simulink model "Controle_UDP_0104"  (R2014a)
settings: Solver=ode45  StartTime=0.0  StopTime=inf  RelTol=1e-3
values from neighbouring files (symbols this model uses):
  in1 = [ 10 10 25 30 0 ] * pi / 180    [data_ACS_HIL.m]
  in2 = [ 0 10 10 30 0 ] * pi / 180    [data_ACS_HIL.m]
  in3 = [ 45 -30 30 30 0 ] * pi / 180    [data_ACS_HIL.m]
  Ixx = I( 1, 1 )    [data_ACS_HIL.m]
  Iyy = I( 2, 2 )    [data_ACS_HIL.m]
  Izz = I( 3, 3 )    [data_ACS_HIL.m]
  J1 = I1 + 3e-06    (= 0.000627567)    [data_ACS_HIL.m]
  J2 = I2 + 3e-06    (= 0.000627567)    [data_ACS_HIL.m]
  J3 = I3 + 3e-06    (= 0.000627567)    [data_ACS_HIL.m]
  Kpx = vp * (wn^2) * Ixx    [data_ACS_HIL.m]
  Kpy = vp * (wn^2) * Iyy    [data_ACS_HIL.m]
  Kpz = vp * (wn^2) * Izz    [data_ACS_HIL.m]
  Krx = vr * 2 * Ixx * wn * qsi    [data_ACS_HIL.m]
  Kry = vr * 2 * Iyy * wn * qsi    [data_ACS_HIL.m]
  Krz = vr * 2 * Izz * wn * qsi    [data_ACS_HIL.m]
  Wx0 = [mW0 0]    [data_ACS_HIL.m]
  Wy0 = [mW0 0]    [data_ACS_HIL.m]
  Wz0 = [mW0 0]    [data_ACS_HIL.m]
libraries: aerolibconvert2 x4, simulink x3, etargetslib x2, instrumentlib x2, xpcutilitieslib x1, slrtlib x1, rtwinlib x1
settings Model: Creator=mayar_000  LastModifiedBy=IMA4BRAZIL
settings DataIOCC: SignalLoggingSaveFormat=ModelDataLogs
settings DebuggingCC: MultiTaskDSMMsg=warning  MultiTaskCondExecSysMsg=none  IntegerOverflowMsg=none  ParameterOverflowMsg=none
settings RTWCC: IncludeERTFirstTime=on

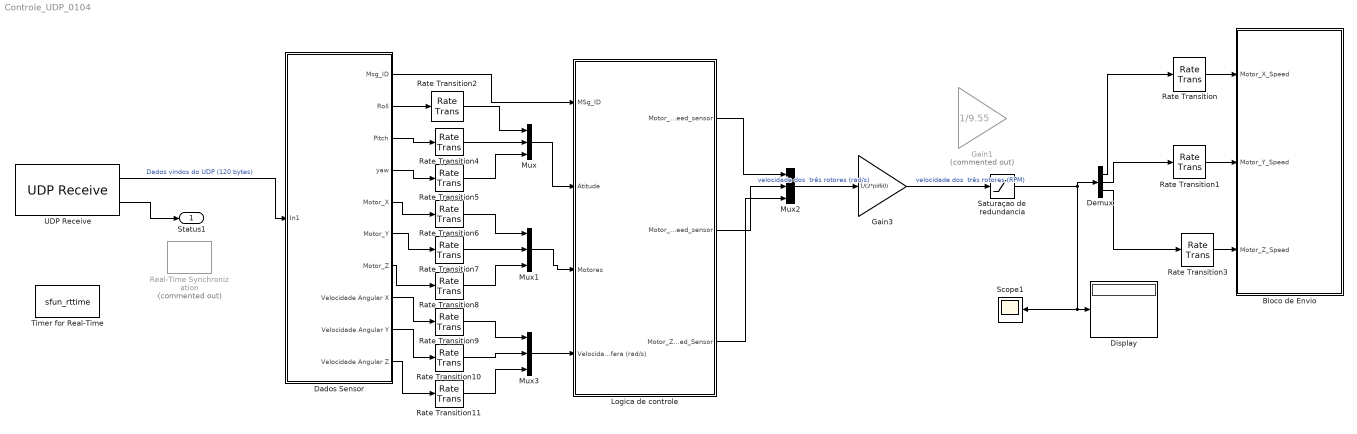
== system Controle_UDP_0104 ==
  Bloco de Envio : Subsystem
      mask Display:
      | port_label('input',1,'\Omega_x','texmode','on')
      | port_label('input',2,'\Omega_y','texmode','on')
      | port_label('input',3,'\Omega_z','texmode','on')
  Dados Sensor : Subsystem
  Demux : Demux  Outputs=3
  Display : Display
  Gain1 : Gain  Commented=on  Gain=1/9.55  SaturateOnIntegerOverflow=on
  Gain3 : Gain  Gain=1/(2*pi/60)
  Logica de controle : Subsystem
  Mux{,1..3} (4 alike) : Mux  Inputs=3
  Rate Transition{,1..11} (12 alike) : RateTransition  OutPortSampleTime=t
  Real-Time Synchronization : rtwinlib/Real-Time Synchronization  Commented=on  SampleTime=0.1  MaxMissedTicks=20  ShowMissedTicks=off  YieldWhenWaiting=off
  Saturaçao de redundancia : Saturate  UpperLimit=4000  LowerLimit=-4000
  Scope1 : Scope
      settings: YMin=-10000  YMax=10000
  Timer for Real-Time : S-Function  FunctionName=sfun_rttime  Parameters=1  EnableBusSupport=off
  UDP Receive : instrumentlib/UDP Receive  Host=172.16.0.62  Port=35204  LocalPort=35204  DataSize=120  EnableBlockingMode=off  Timeout=50  SampleTime=0.25  DataType=uint8  ByteOrder=BigEndian
  Status1 : Outport
  wires:
  UDP Receive/2 -> Status1/1
  UDP Receive/1 -> Dados Sensor/1(In1)  "Dados vindos do UDP (120 bytes)"
  Rate Transition/1 -> Bloco de Envio/1(Motor_X_Speed)
  Rate Transition1/1 -> Bloco de Envio/2(Motor_Y_Speed)
  Demux/1 -> Rate Transition/1
  Demux/2 -> Rate Transition1/1
  Demux/3 -> Rate Transition3/1
  Rate Transition3/1 -> Bloco de Envio/3(Motor_Z_Speed)
  Dados Sensor/1(Msg_ID) -> Logica de controle/1(MSg_ID)
  Mux/1 -> Logica de controle/2(Atitude)
  Mux1/1 -> Logica de controle/3(Motores)
  Logica de controle/1(Motor_X_Speed_sensor) -> Mux2/1
  Logica de controle/2(Motor_Y_Speed_sensor) -> Mux2/2
  Logica de controle/3(Motor_Z_Speed_Sensor) -> Mux2/3
  Dados Sensor/2(Roll) -> Rate Transition2/1
  Dados Sensor/3(Pitch) -> Rate Transition4/1
  Dados Sensor/4(yaw) -> Rate Transition5/1
  Dados Sensor/7(Motor_Z) -> Rate Transition8/1
  Dados Sensor/6(Motor_Y) -> Rate Transition7/1
  Dados Sensor/5(Motor_X) -> Rate Transition6/1
  Rate Transition2/1 -> Mux/1
  Rate Transition4/1 -> Mux/2
  Rate Transition5/1 -> Mux/3
  Rate Transition6/1 -> Mux1/1
  Rate Transition7/1 -> Mux1/2
  Rate Transition8/1 -> Mux1/3
  Saturaçao de redundancia/1 -> Demux/1, Scope1/1, Display/1
  Mux2/1 -> Gain3/1  "velocidade dos  três rotores (rad/s)"
  Gain3/1 -> Saturaçao de redundancia/1  "velocidade dos  três rotores (RPM)"
  Dados Sensor/8(Velocidade Angular X) -> Rate Transition9/1
  Dados Sensor/9(Velocidade Angular Y) -> Rate Transition10/1
  Dados Sensor/10(Velocidade Angular Z) -> Rate Transition11/1
  Mux3/1 -> Logica de controle/4(Velocidade Angular da Esfera (rad/s))
  Rate Transition9/1 -> Mux3/1
  Rate Transition10/1 -> Mux3/2
  Rate Transition11/1 -> Mux3/3

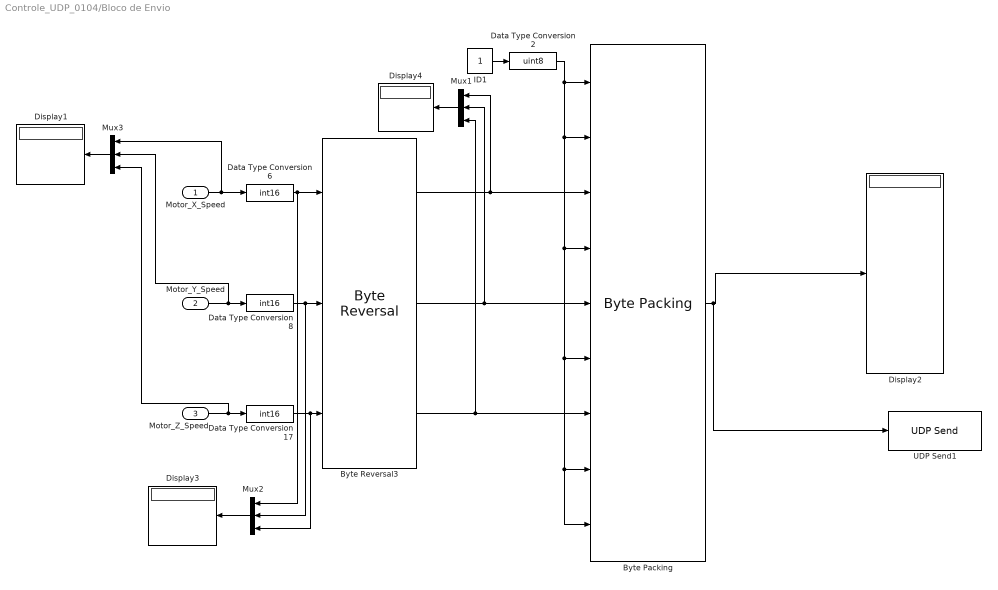
== system Controle_UDP_0104/Bloco de Envio ==
  Motor_X_Speed : Inport
  Motor_Y_Speed : Inport  Port=2
  Motor_Z_Speed : Inport  Port=3
  "Byte Packing " : xpcutilitieslib/Byte Packing   MaskPackedDataType=uint8  MaskUnpackedDataTypes={'uint8','uint8','int16','uint8','int16','uint8','int16','uint8', 'uint8'}  MaskAlignment=1
  Byte Reversal3 : etargetslib/Byte Reversal  numInp=3
  Data Type Conversion17 : DataTypeConversion  OutDataTypeStr=int16  SaturateOnIntegerOverflow=on
  Data Type Conversion2 : DataTypeConversion  OutDataTypeStr=uint8  SaturateOnIntegerOverflow=on
  Data Type Conversion6 : DataTypeConversion  OutDataTypeStr=int16  SaturateOnIntegerOverflow=on
  Data Type Conversion8 : DataTypeConversion  OutDataTypeStr=int16  SaturateOnIntegerOverflow=on
  Display{1..4} (4 alike) : Display
      Display3 settings: Format=hex (Stored Integer)
      Display4 settings: Format=hex (Stored Integer)
  ID1 : Constant  OutDataTypeStr=uint8
  Mux1 : Mux  Inputs=3
  Mux2 : Mux  Inputs=3
  Mux3 : Mux  Inputs=3
  UDP Send1 : instrumentlib/UDP Send  Host=172.16.0.62  Port=35308  LocalPort=-1  EnableBlockingMode=off  ByteOrder=LittleEndian
  wires:
  Motor_Y_Speed/1 -> Mux3/2, Data Type Conversion8/1
  Data Type Conversion6/1 -> Mux2/1, Byte Reversal3/1
  Motor_X_Speed/1 -> Mux3/1, Data Type Conversion6/1
  "Byte Packing "/1 -> Display2/1, UDP Send1/1
  Data Type Conversion8/1 -> Mux2/2, Byte Reversal3/2
  Data Type Conversion17/1 -> Mux2/3, Byte Reversal3/3
  Byte Reversal3/2 -> Mux1/2, "Byte Packing "/5
  Data Type Conversion2/1 -> "Byte Packing "/9, "Byte Packing "/8, "Byte Packing "/6, "Byte Packing "/4, "Byte Packing "/2, "Byte Packing "/1
  ID1/1 -> Data Type Conversion2/1
  Byte Reversal3/1 -> Mux1/1, "Byte Packing "/3
  Mux3/1 -> Display1/1
  Mux1/1 -> Display4/1
  Byte Reversal3/3 -> Mux1/3, "Byte Packing "/7
  Motor_Z_Speed/1 -> Mux3/3, Data Type Conversion17/1
  Mux2/1 -> Display3/1

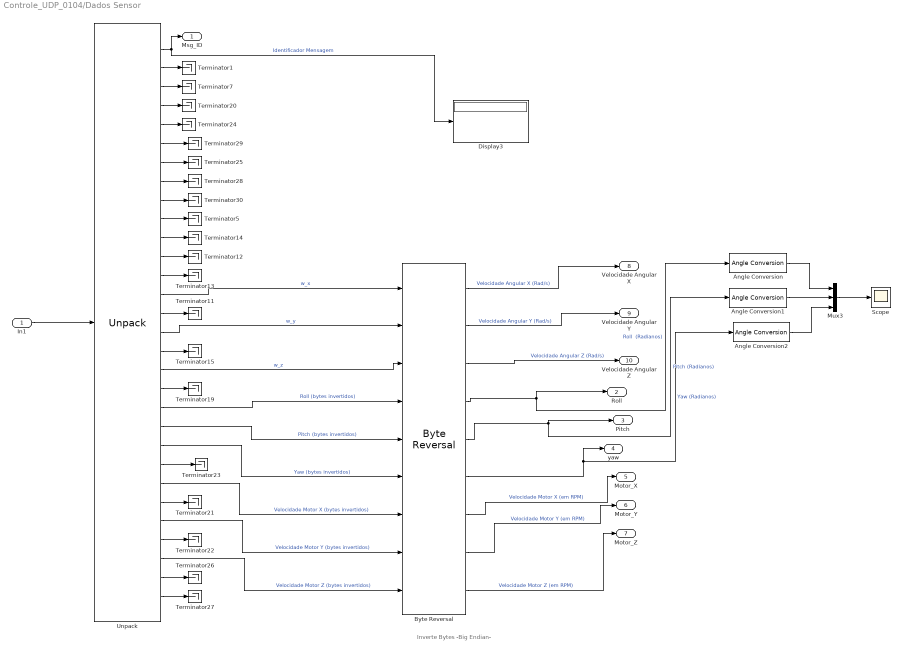
== system Controle_UDP_0104/Dados Sensor ==
  note: Inverte Bytes
      | -Big Endian-
  In1 : Inport
  Angle Conversion : aerolibconvert2/Angle Conversion  IU=rad  OU=deg
  Angle Conversion1 : aerolibconvert2/Angle Conversion  IU=rad  OU=deg
  Angle Conversion2 : aerolibconvert2/Angle Conversion  IU=rad  OU=deg
  Byte Reversal : etargetslib/Byte Reversal  numInp=9
  Display3 : Display
  Mux3 : Mux  Inputs=3
  Scope : Scope
      settings: YMin=-10  YMax=100  SaveName=ScopeData2
  Terminator{1,5,7,11..15,19..30} (20 alike) : Terminator
  Unpack : slrtlib/UDP/Unpack   dimensions={[1,1],[1,1],[1,1],[1,1],[1,1],[1,1],[1,1],[1,1],[1,1],[1,1],[1,1],[1,1],[1,1],[1,1],[1,1],[1,1],[1,1],[1,1],[1,1],[1,1],[1,1],[1,1],[1,4],[1,1],[1,1],[1,1],[1,1],[1,1],[1,1],[1,1]}  datatypes={'uint8','single','uint32','single','uint32','single','uint32','single','uint32','single','uint32','single','uint32','single','uint32','single','uint32','single','uint32','single','single','single','single','int16','uint32','int16','uint32','int16','uint32','uint8'}  byteAlign=1
  Msg_ID : Outport
  Roll : Outport  Port=2
  Pitch : Outport  Port=3
  yaw : Outport  Port=4
  Motor_X : Outport  Port=5
  Motor_Y : Outport  Port=6
  Motor_Z : Outport  Port=7
  Velocidade Angular X : Outport  Port=8
  Velocidade Angular Y : Outport  Port=9
  Velocidade Angular Z : Outport  Port=10
  wires:
  Unpack/4 -> Terminator20/1
  Unpack/5 -> Terminator24/1
  Unpack/6 -> Terminator29/1
  Unpack/3 -> Terminator7/1
  Byte Reversal/8 -> Motor_Y/1  "Velocidade Motor Y (em RPM)"
  Unpack/1 -> Msg_ID/1, Display3/1  "Identificador Mensagem"
  Unpack/2 -> Terminator1/1
  Unpack/7 -> Terminator25/1
  Unpack/8 -> Terminator28/1
  Byte Reversal/5 -> Pitch/1, Angle Conversion1/1  "Pitch (Radianos)"
  Byte Reversal/7 -> Motor_X/1  "Velocidade Motor X (em RPM)"
  Unpack/28 -> Byte Reversal/9  "Velocidade Motor Z (bytes invertidos)"
  Unpack/19 -> Terminator19/1
  Unpack/11 -> Terminator14/1
  Unpack/14 -> Byte Reversal/1  "w_x"
  Unpack/16 -> Byte Reversal/2  "w_y"
  Unpack/30 -> Terminator27/1
  Unpack/20 -> Byte Reversal/4  "Roll (bytes invertidos)"
  Unpack/21 -> Byte Reversal/5  "Pitch (bytes invertidos)"
  Unpack/12 -> Terminator12/1
  Unpack/23 -> Terminator23/1
  Unpack/18 -> Byte Reversal/3  "w_z"
  Unpack/27 -> Terminator22/1
  Unpack/25 -> Terminator21/1
  Unpack/15 -> Terminator11/1
  Unpack/13 -> Terminator13/1
  Unpack/10 -> Terminator5/1
  Unpack/9 -> Terminator30/1
  Unpack/17 -> Terminator15/1
  Unpack/22 -> Byte Reversal/6  "Yaw (bytes invertidos)"
  Unpack/24 -> Byte Reversal/7  "Velocidade Motor X (bytes invertidos)"
  Unpack/26 -> Byte Reversal/8  "Velocidade Motor Y (bytes invertidos)"
  Unpack/29 -> Terminator26/1
  Byte Reversal/4 -> Roll/1, Angle Conversion/1  "Roll  (Radianos)"
  Byte Reversal/9 -> Motor_Z/1  "Velocidade Motor Z (em RPM)"
  Byte Reversal/6 -> yaw/1, Angle Conversion2/1  "Yaw (Radianos)"
  In1/1 -> Unpack/1
  Angle Conversion/1 -> Mux3/1
  Angle Conversion1/1 -> Mux3/2
  Angle Conversion2/1 -> Mux3/3
  Mux3/1 -> Scope/1
  Byte Reversal/3 -> Velocidade Angular Z/1  "Velocidade Angular Z (Rad/s)"
  Byte Reversal/2 -> Velocidade Angular Y/1  "Velocidade Angular Y (Rad/s)"
  Byte Reversal/1 -> Velocidade Angular X/1  "Velocidade Angular X (Rad/s)"

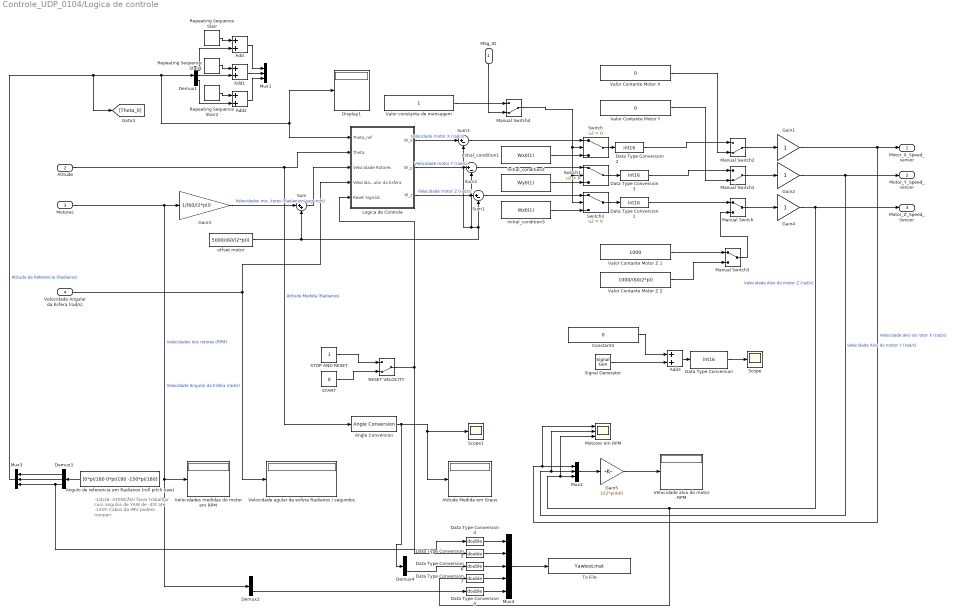
== system Controle_UDP_0104/Logica de controle ==
  note: -1/4/16-
      | ATENÇÃO!
      |
      | favor trabalhar com
      | angulos de YAW de
      | -45º até -135º!
      | Cabos da IMU podem romper!
  MSg_ID : Inport
  Atitude : Inport  Port=2
  Motores : Inport  Port=3
  Velocidade Angular da Esfera (rad/s) : Inport  Port=4
  Add{,1..3} (4 alike) : Sum
  Angle Conversion : aerolibconvert2/Angle Conversion  IU=rad  OU=deg
  Angulo de referencia em Radianos (roll pitch yaw) : Constant  Value=[0*pi/180 0*pi/180 -150*pi/180]
  Atitude Medida em Graus : Display
      settings: Decimation=3
  Constant3 : Constant  Value=0  OutDataTypeStr=int16
  Data Type Conversion : DataTypeConversion  OutDataTypeStr=int16
  Data Type Conversion1 : DataTypeConversion  OutDataTypeStr=int16  SaturateOnIntegerOverflow=on
  Data Type Conversion2 : DataTypeConversion  OutDataTypeStr=int16  SaturateOnIntegerOverflow=on
  Data Type Conversion3 : DataTypeConversion  OutDataTypeStr=int16  SaturateOnIntegerOverflow=on
  Data Type Conversion{4..8} (5 alike) : DataTypeConversion  OutDataTypeStr=double  SaturateOnIntegerOverflow=on
  Demux{1..4} (4 alike) : Demux  Outputs=3
  Display1 : Display
  Gain1 : Gain  OutDataTypeStr=int16  SaturateOnIntegerOverflow=on
  Gain2 : Gain  OutDataTypeStr=int16  SaturateOnIntegerOverflow=on
  Gain3 : Gain  Gain=1/(60/(2*pi))
  Gain4 : Gain  OutDataTypeStr=int16  SaturateOnIntegerOverflow=on
  Gain5 : Gain  Gain=1/(2*pi/60)  OutDataTypeStr=int16  SaturateOnIntegerOverflow=on
  Initial_condition1 : Constant  Value=Wx0(1)  OutDataTypeStr=int16
  Initial_condition2 : Constant  Value=Wy0(1)  OutDataTypeStr=int16
  Initial_condition3 : Constant  Value=Wz0(1)  OutDataTypeStr=int16
  Logica de Controle : Subsystem
      mask Display:
      | port_label('input',1,'\theta^{ref}','texmode','on')
      | port_label('input',2,'\theta','texmode','on')
      | port_label('input',3,'\Omega','texmode','on')
      | port_label('input',4,'\omega','texmode','on')
      | port_label('input',5,'RESET','texmode','on')
      | 
      | port_label('output',1,'\Omega_{x}^{des}','texmode','on')
      | port_label('output',2,'\Omega_{y}^{des}','texmode','on')
      | port_label('output',3,'\Omega_{z}^{des}','texmode','on')
  Manual Switch : ManualSwitch
  Manual Switch1 : ManualSwitch  CurrentSetting=0
  Manual Switch2 : ManualSwitch  CurrentSetting=0
  Manual Switch3 : ManualSwitch
  Manual Switch4 : ManualSwitch  CurrentSetting=0
  Motores em RPM : Scope  NumInputPorts=3
      settings: YMin=0~-5~-5  YMax=1000~5~5  SaveName=sinal_referencia2
  Mux1 : Mux  Inputs=3
  Mux2 : Mux  Inputs=3
  Mux3 : Mux  Inputs=3
  Mux4 : Mux  Inputs=5
  RESET VELOCITY : ManualSwitch  CurrentSetting=0
  Repeating Sequence Stair : simulink/Sources/Repeating Sequence Stair  OutValues=in1.'  tsamp=1000  OutMin=[]  OutMax=[]  OutDataTypeStr=double  OutputDataTypeScalingMode=double  OutDataType=fixdt(0,8)  ConRadixGroup=Best Precision: Vector-wise  OutScaling=2^-12
  Repeating Sequence Stair1 : simulink/Sources/Repeating Sequence Stair  OutValues=in2.'  tsamp=1000  OutMin=[]  OutMax=[]  OutDataTypeStr=double  OutputDataTypeScalingMode=double  OutDataType=fixdt(0,8)  ConRadixGroup=Best Precision: Vector-wise  OutScaling=2^-12
  Repeating Sequence Stair2 : simulink/Sources/Repeating Sequence Stair  OutValues=in3.'  tsamp=1000  OutMin=[]  OutMax=[]  OutDataTypeStr=double  OutputDataTypeScalingMode=double  OutDataType=fixdt(0,8)  ConRadixGroup=Best Precision: Vector-wise  OutScaling=2^-12
  START : Constant  Value=0  OutDataTypeStr=boolean
  STOP AND RESET : Constant  OutDataTypeStr=boolean
  Scope : Scope
      settings: YMin=-1050  YMax=-950  SaveName=sinal_referencia
  Scope1 : Scope
      settings: YMin=-175  YMax=25  SaveName=ScopeData4
  Signal Generator : SignalGenerator  WaveForm=square  Amplitude=1000  Frequency=0.1
  Sum : Sum  Inputs=|++
  Sum1 : Sum  Inputs=|+-
  Sum2 : Sum  Inputs=|+-
  Sum3 : Sum  Inputs=|+-
  Switch : Switch  Criteria=u2 > Threshold  OutDataTypeStr=int16
  Switch1 : Switch  Criteria=u2 > Threshold  OutDataTypeStr=int16
  Switch3 : Switch  Criteria=u2 > Threshold  OutDataTypeStr=int16
  To File : ToFile  Filename=Yawtest.mat  MatrixName=test_var
  Valor Contante Motor X : Constant  Value=0  OutDataTypeStr=int16
  Valor Contante Motor Y : Constant  Value=0  OutDataTypeStr=int16
  Valor Contante Motor Z 1 : Constant  Value=1000  OutDataTypeStr=int16
  Valor Contante Motor Z 2 : Constant  Value=1000/(60/2*pi)  OutDataTypeStr=int16
  Valor constante de mensagem : Constant  OutDataTypeStr=int16
  Velocidade agular da esfera Radianos / segundos : Display
      settings: Format=decimal (Stored Integer)  Decimation=3
  Velocidade alvo do motor RPM : Display
      settings: Decimation=3
  Velocidades medidas do motor em RPM : Display
      settings: Decimation=3
  offset motor : Constant  Value=5000/(60/(2*pi))  OutDataTypeStr=boolean
  Motor_X_Speed_sensor : Outport
  Motor_Y_Speed_sensor : Outport  Port=2
  Motor_Z_Speed_Sensor : Outport  Port=3  OutDataTypeStr=int16
  wires:
  Add1/1 -> Mux1/2
  Demux1/1 -> Add/2
  Add2/1 -> Mux1/3
  Mux3/1 -> Logica de Controle/1(Theta_ref), Display1/1, Demux1/1, [Theta_0]  "Atitude de Referencia (Radianos)"
  Demux1/2 -> Add1/2
  Repeating Sequence Stair/1 -> Add/1
  Repeating Sequence Stair2/1 -> Add2/1
  Repeating Sequence Stair1/1 -> Add1/1
  Demux1/3 -> Add2/2
  Add/1 -> Mux1/1
  Initial_condition1/1 -> Switch/3
  Motores/1 -> Demux2/1, Velocidades medidas do motor em RPM/1, Gain3/1  "Velocidades dos rotores (RPM)"
  Initial_condition2/1 -> Switch1/3
  Logica de Controle/1(W_x) -> Sum3/1  "Velocidade motor X (rad/s)"
  Logica de Controle/2(W_y) -> Sum2/1  "Velocidade motor Y (rad/s)"
  Logica de Controle/3(W_z) -> Sum1/1  "Velocidade motor Z (rad/s)"
  Switch/1 -> Data Type Conversion2/1
  Data Type Conversion/1 -> Scope/1
  Initial_condition3/1 -> Switch3/3
  Signal Generator/1 -> Add3/2
  Constant3/1 -> Add3/1
  Add3/1 -> Data Type Conversion/1
  Switch3/1 -> Data Type Conversion1/1
  Data Type Conversion1/1 -> Manual Switch/1
  Switch1/1 -> Data Type Conversion3/1
  Data Type Conversion2/1 -> Manual Switch2/1
  Data Type Conversion3/1 -> Manual Switch1/1
  Valor Contante Motor Y/1 -> Manual Switch1/2
  Valor Contante Motor X/1 -> Manual Switch2/2
  Gain3/1 -> Sum/1  "Velocidades motores (Radianos / segundo)"
  Manual Switch/1 -> Gain4/1
  Manual Switch1/1 -> Gain2/1
  Manual Switch2/1 -> Gain1/1
  Gain1/1 -> Motores em RPM/1, Mux2/1, Motor_X_Speed_sensor/1  "Velocidade alvo do rotor X (rad/s)"
  Gain2/1 -> Motores em RPM/2, Mux2/2, Motor_Y_Speed_sensor/1  "Velocidade Alvo do motor Y (rad/s)"
  Gain4/1 -> Data Type Conversion7/1, Motores em RPM/3, Mux2/3, Motor_Z_Speed_Sensor/1  "Velocidade Alvo do motor Z (rad/s)"
  Atitude/1 -> Logica de Controle/2(Theta), Angle Conversion/1  "Atitude Medida (Radianos)"
  Valor Contante Motor Z 1/1 -> Manual Switch3/1
  Valor Contante Motor Z 2/1 -> Manual Switch3/2
  Manual Switch3/1 -> Manual Switch/2
  Valor constante de mensagem/1 -> Manual Switch4/1
  MSg_ID/1 -> Manual Switch4/2
  Manual Switch4/1 -> Switch3/2, Switch1/2, Switch/2
  STOP AND RESET/1 -> RESET VELOCITY/1
  START/1 -> RESET VELOCITY/2
  Mux2/1 -> Gain5/1
  Gain5/1 -> Velocidade alvo do motor RPM/1
  Sum/1 -> Logica de Controle/3(Velocidade Rotores)
  offset motor/1 -> Sum3/2, Sum2/2, Sum1/2, Sum/2
  Sum3/1 -> Switch/1
  Sum2/1 -> Switch1/1
  Sum1/1 -> Switch3/1
  Velocidade Angular da Esfera (rad/s)/1 -> Logica de Controle/4(Velocidade Angular da Esfera), Velocidade agular da esfera Radianos / segundos/1  "Velocidade Angular da Esfera (rad/s)"
  Demux3/3 -> Data Type Conversion4/1, Mux3/3
  Demux3/2 -> Mux3/2
  Demux3/1 -> Mux3/1
  Angulo de referencia em Radianos (roll pitch yaw)/1 -> Demux3/1
  Angle Conversion/1 -> Demux4/1, Atitude Medida em Graus/1, Scope1/1
  Demux4/3 -> Data Type Conversion6/1
  Mux4/1 -> To File/1
  Demux2/3 -> Data Type Conversion8/1
  RESET VELOCITY/1 -> Data Type Conversion5/1, Logica de Controle/5(Reset Signal1)
  Data Type Conversion4/1 -> Mux4/1
  Data Type Conversion5/1 -> Mux4/2
  Data Type Conversion6/1 -> Mux4/3
  Data Type Conversion7/1 -> Mux4/4
  Data Type Conversion8/1 -> Mux4/5

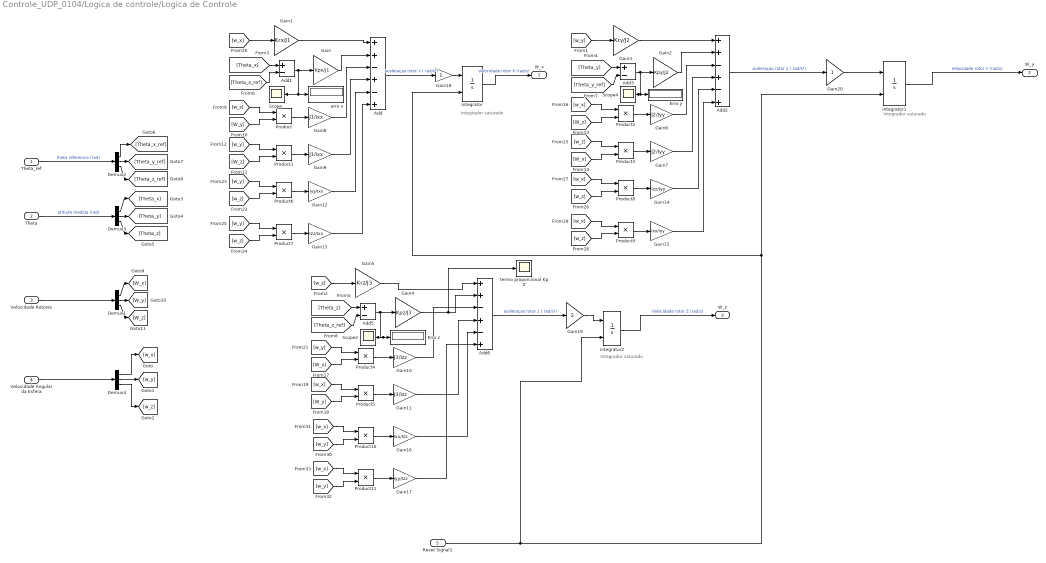
== system Controle_UDP_0104/Logica de controle/Logica de Controle ==
  note: Integrador
      | saturado
  note: Integrador
      | saturado
  note: Integrador
      | saturado
  Theta_ref : Inport
  Theta : Inport  Port=2
  Velocidade Rotores : Inport  Port=3
  Velocidade Angular da Esfera : Inport  Port=4
  Reset Signal1 : Inport  Port=5
  Add : Sum  Inputs=++-+-+
  Add1 : Sum  Inputs=+-
  Add2 : Sum  Inputs=++-+-+
  Add3 : Sum  Inputs=+-
  Add5 : Sum  Inputs=+-
  Add6 : Sum  Inputs=++-+-+
  Demux{1..4} (4 alike) : Demux  Outputs=3
  Erro y : Display
  Erro z : Display
  Gain : Gain  Gain=Kpx/J1
  Gain1 : Gain  Gain=Krx/J1
  Gain10 : Gain  Gain=J3/Izz
  Gain11 : Gain  Gain=J3/Izz
  Gain12 : Gain  Gain=Iyy/Ixx
  Gain13 : Gain  Gain=Izz/Ixx
  Gain14 : Gain  Gain=Izz/Iyy
  Gain15 : Gain  Gain=Ixx/Iyy
  Gain16 : Gain  Gain=Ixx/Izz
  Gain17 : Gain  Gain=Iyy/Izz
  Gain18 : Gain  SaturateOnIntegerOverflow=on
  Gain19 : Gain  Gain=2  SaturateOnIntegerOverflow=on
  Gain2 : Gain  Gain=Kpy/J2
  Gain20 : Gain  SaturateOnIntegerOverflow=on
  Gain3 : Gain  Gain=Kry/J2
  Gain4 : Gain  Gain=Kpz/J3
  Gain5 : Gain  Gain=Krz/J3
  Gain6 : Gain  Gain=J2/Iyy
  Gain7 : Gain  Gain=J2/Iyy
  Gain8 : Gain  Gain=J1/Ixx
  Gain9 : Gain  Gain=J1/Ixx
  Integrator : Integrator  ExternalReset=level  InitialCondition=Wx0(1)  LimitOutput=on  UpperSaturationLimit=4500*2*pi/60  LowerSaturationLimit=-4500*2*pi/60
  Integrator1 : Integrator  ExternalReset=level  InitialCondition=Wy0(1)  LimitOutput=on  UpperSaturationLimit=4500*2*pi/60  LowerSaturationLimit=-4000*2*pi/60
  Integrator2 : Integrator  ExternalReset=level  InitialCondition=Wz0(1)  LimitOutput=on  UpperSaturationLimit=4500*2*pi/60  LowerSaturationLimit=-4500*2*pi/60
  Product{,1..11} (12 alike) : Product  RndMeth=Zero
  Scope : Scope
      settings: TimeRange=2  YMin=-0.8  YMax=0.6000000000000001  SaveName=ErroX
  Scope2 : Scope
      settings: YMin=-0.33  YMax=-0.2  SaveName=ScopeData3
  Scope4 : Scope
      settings: TimeRange=2  YMin=-0.35  YMax=0  SaveName=ScopeData5
  erro x : Display
  termo proporcional Kp Z : Scope
      settings: YMin=-2.25  YMax=1.25  SaveName=ScopeData7
  W_x : Outport
  W_y : Outport  Port=2
  W_z : Outport  Port=3
  wires:
  [w_x] -> Gain1/1
  Add1/1 -> Gain/1, erro x/1, Scope/1
  [w_y] -> Gain3/1
  Add3/1 -> Gain2/1, Scope4/1, Erro y/1
  [w_z] -> Gain5/1
  Add2/1 -> Gain20/1  "aceleraçao rotor y ( rad/s²)"
  Gain1/1 -> Add/1
  Gain/1 -> Add/2
  [Theta_x] -> Add1/1
  [Theta_x_ref] -> Add1/2
  Gain2/1 -> Add2/2
  Gain3/1 -> Add2/1
  [Theta_y] -> Add3/1
  [Theta_y_ref] -> Add3/2
  Gain5/1 -> Add6/1
  Gain4/1 -> termo proporcional Kp Z/1, Add6/2
  [Theta_z] -> Add5/1
  [Theta_z_ref] -> Add5/2
  Velocidade Rotores/1 -> Demux1/1
  Theta_ref/1 -> Demux2/1  "theta referencia (rad)"
  Demux1/1 -> [W_x]
  Demux1/2 -> [W_y]
  Demux1/3 -> [W_z]
  Demux3/1 -> [Theta_x]
  Demux3/2 -> [Theta_y]
  Demux3/3 -> [Theta_z]
  Demux2/1 -> [Theta_x_ref]
  Demux2/2 -> [Theta_y_ref]
  Demux2/3 -> [Theta_z_ref]
  [w_z] -> Product/1
  [W_y] -> Product/2
  Product/1 -> Gain8/1
  [w_y] -> Product1/1
  [W_z] -> Product1/2
  Product1/1 -> Gain9/1
  [w_x] -> Product2/1
  [W_z] -> Product2/2
  Product2/1 -> Gain6/1
  [w_z] -> Product3/1
  [W_x] -> Product3/2
  Product3/1 -> Gain7/1
  [w_y] -> Product4/1
  [W_x] -> Product4/2
  Product4/1 -> Gain10/1
  [w_x] -> Product5/1
  [W_y] -> Product5/2
  Product5/1 -> Gain11/1
  Gain6/1 -> Add2/3
  Gain7/1 -> Add2/4
  Gain8/1 -> Add/3
  Gain9/1 -> Add/4
  [w_y] -> Product6/1
  [w_z] -> Product6/2
  Product6/1 -> Gain12/1
  Gain12/1 -> Add/5
  [w_y] -> Product7/1
  [w_z] -> Product7/2
  Product7/1 -> Gain13/1
  [w_x] -> Product8/1
  [w_z] -> Product8/2
  Product8/1 -> Gain14/1
  [w_x] -> Product9/1
  [w_z] -> Product9/2
  Product9/1 -> Gain15/1
  Gain14/1 -> Add2/5
  Gain15/1 -> Add2/6
  [w_x] -> Product10/1
  [w_y] -> Product10/2
  Product10/1 -> Gain16/1
  [w_x] -> Product11/1
  [w_y] -> Product11/2
  Product11/1 -> Gain17/1
  Gain10/1 -> Add6/3
  Gain11/1 -> Add6/4
  Gain16/1 -> Add6/5
  Gain17/1 -> Add6/6
  Add6/1 -> Gain19/1  "aceleraçao rotor z ( rad/s²)"
  Gain13/1 -> Add/6
  Add/1 -> Gain18/1  "aceleraçao rotor x ( rad/s²)"
  Add5/1 -> Scope2/1, Erro z/1, Gain4/1
  Integrator/1 -> W_x/1  "Velocidade rotor X (rad/s)"
  Integrator2/1 -> W_z/1  "Velocidade rotor Z (rad/s)"
  Integrator1/1 -> W_y/1  "Velocidade rotor Y (rad/s)"
  Theta/1 -> Demux3/1  "atitude medida (rad)"
  Reset Signal1/1 -> Integrator2/2, Integrator/2, Integrator1/2
  Gain19/1 -> Integrator2/1
  Gain20/1 -> Integrator1/1
  Gain18/1 -> Integrator/1
  Velocidade Angular da Esfera/1 -> Demux4/1
  Demux4/2 -> [w_y]
  Demux4/1 -> [w_x]
  Demux4/3 -> [w_z]
